simulink model "LQR"  (R2020a)
settings: Solver=VariableStepAuto  StartTime=0.0  StopTime=20  RelTol=1e-3
values from neighbouring files (symbols this model uses):
  A = stateSpaceModel.A    [System_Control.m]    (also in script2.m)
  B = stateSpaceModel.B    [System_Control.m]    (also in script2.m)
  C = stateSpaceModel.C    [System_Control.m]    (also in script2.m)
  Ts = stateSpaceModel.Ts    [System_Control.m]    (also in script2.m)
undefined symbols (not defined in the file or in its folder): K
settings Model: Creator=Gil  LastModifiedBy=Gil
settings DebuggingCC: ArithmeticOperatorsInVariantConditions=warning
settings SFSimCC: CustomCodeUndefinedFunction=UseInterfaceOnly

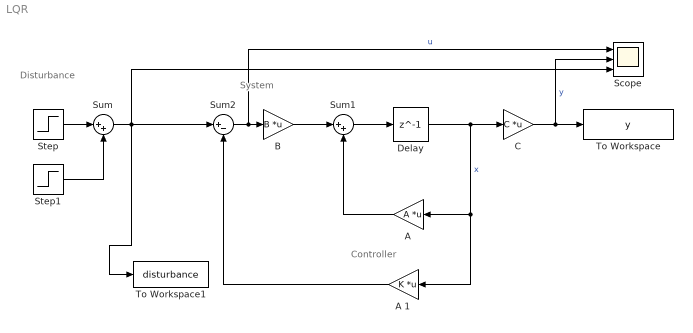
== system LQR ==
  note: Controller
  note: System
  note: Disturbance
  "A " : Gain  Gain=A  Multiplication=Matrix(K*u)
  A 1 : Gain  Gain=K  Multiplication=Matrix(K*u)
  B : Gain  Gain=B  Multiplication=Matrix(K*u)
  C : Gain  Gain=C  Multiplication=Matrix(K*u)
  Delay : Delay  DelayLength=1  InitialCondition=0  SampleTime=Ts
  Scope : Scope  NumInputPorts=3
  Step : Step  Time=2  Before=-1  SampleTime=Ts
  Step1 : Step  Time=4  Before=1  After=-1  SampleTime=Ts
  Sum : Sum  Inputs=|++
  Sum1 : Sum  Inputs=|++
  Sum2 : Sum  Inputs=|+-
  To Workspace : ToWorkspace  VariableName=y  SaveFormat=Structure With Time  SampleTime=Ts
  To Workspace1 : ToWorkspace  VariableName=disturbance  SaveFormat=Structure With Time  SampleTime=Ts
  wires:
  B/1 -> Sum1/1
  Delay/1 -> A 1/1, "A "/1, C/1  "x"
  "A "/1 -> Sum1/2
  Sum1/1 -> Delay/1
  C/1 -> Scope/2, To Workspace/1  "y"
  Step1/1 -> Sum/2
  Step/1 -> Sum/1
  Sum2/1 -> Scope/1, B/1  "u"
  A 1/1 -> Sum2/2
  Sum/1 -> Sum2/1, To Workspace1/1, Scope/3
